simulink model "dynamik"  (R2016b)
settings: Solver=ode23s  StartTime=0.0  StopTime=100  RelTol=1e-3
values from neighbouring files (symbols this model uses):
  L = T-V    [modeldynamik.m]
undefined symbols (not defined in the file or in its folder): a_acc, a_de, dot_phi_soll, I_R, l, m, Mass
libraries: simulink x3
settings Model: Creator=Alexa  LastModifiedBy=Alexa

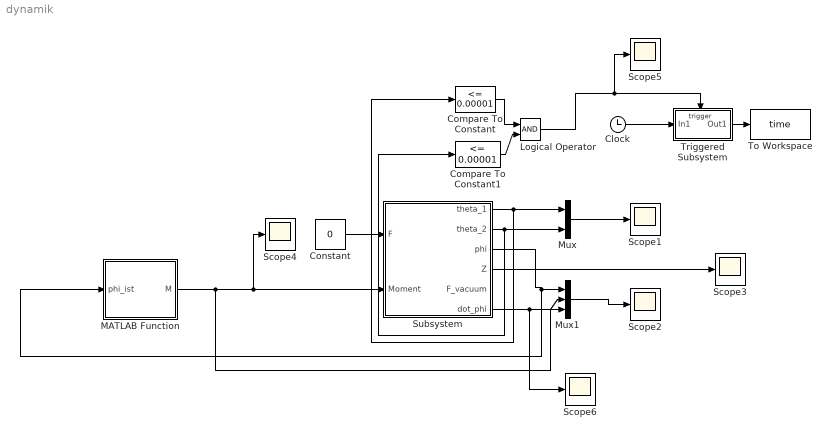
== system dynamik ==
  Clock : Clock
  Compare To Constant : simulink/Logic and Bit Operations/Compare To Constant  relop=<=  const=0.00001  OutDataTypeStr=boolean
  Compare To Constant1 : simulink/Logic and Bit Operations/Compare To Constant  relop=<=  const=0.00001  OutDataTypeStr=boolean
  Constant : Constant  Value=0
  Logical Operator : Logic  AllPortsSameDT=off  OutDataTypeStr=boolean
  MATLAB Function : MATLAB Function  TreatAsAtomicUnit=on
  Mux : Mux  Inputs=2
  Mux1 : Mux  Inputs=3
  Scope{1..6} (6 alike) : Scope
  Subsystem : Subsystem
  To Workspace : ToWorkspace  VariableName=time  SaveFormat=Timeseries  SampleTime=-1
  Triggered Subsystem : Subsystem  TreatAsAtomicUnit=on
  wires:
  Subsystem/1(theta_1) -> Compare To Constant/1, Mux/1
  Subsystem/2(theta_2) -> Compare To Constant1/1, Mux/2
  Mux/1 -> Scope1/1
  Subsystem/6(dot_phi) -> Scope6/1, Mux1/2
  Constant/1 -> Subsystem/1(F)
  Subsystem/3(phi) -> MATLAB Function/1(phi_ist), Mux1/1
  Mux1/1 -> Scope2/1
  Subsystem/4(Z) -> Scope3/1
  Clock/1 -> Triggered Subsystem/1(In1)
  Compare To Constant/1 -> Logical Operator/1
  Compare To Constant1/1 -> Logical Operator/2
  Logical Operator/1 -> Scope5/1, Triggered Subsystem/Trigger
  Triggered Subsystem/1(Out1) -> To Workspace/1
  MATLAB Function/1(M) -> Mux1/3, Subsystem/2(Moment), Scope4/1

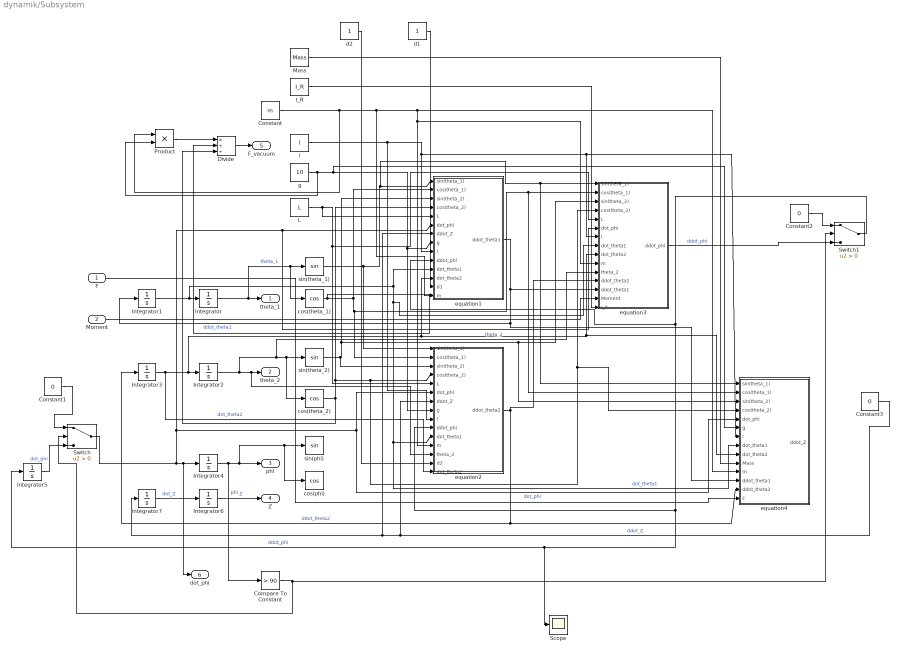
== system dynamik/Subsystem ==
  F : Inport
  Moment : Inport  Port=2
  Compare To Constant : simulink/Logic and Bit Operations/Compare To Constant  relop=>  const=90  OutDataTypeStr=boolean
  Constant : Constant  Value=m
  Constant1 : Constant  Value=0
  Constant2 : Constant  Value=0
  Constant3 : Constant  Value=0
  Divide : Product  Inputs=*//
  I_R : Constant  Value=I_R
  Integrator{,1..7} (8 alike) : Integrator
  L : Constant  Value=L
  Mass : Constant  Value=Mass
  Product : Product
  Scope : Scope
  Switch : Switch  Criteria=u2 > Threshold
  Switch1 : Switch  Criteria=u2 > Threshold
  cos(phi) : Trigonometry  Operator=cos
  cos(theta_1) : Trigonometry  Operator=cos
  cos(theta_2) : Trigonometry  Operator=cos
  d1 : Constant
  d2 : Constant
  equation1 : Subsystem
  equation2 : Subsystem
  equation3 : Subsystem
  equation4 : Subsystem
  g : Constant  Value=10
  l : Constant  Value=l
  sin(phi) : Trigonometry
  sin(theta_1) : Trigonometry
  sin(theta_2) : Trigonometry
  theta_1 : Outport
  theta_2 : Outport  Port=2
  phi : Outport  Port=3
  Z : Outport  Port=4
  F_vacuum : Outport  Port=5
  dot_phi : Outport  Port=6
  wires:
  Integrator/1 -> cos(theta_1)/1, sin(theta_1)/1, theta_1/1  "theta_1"
  Integrator1/1 -> equation1/11(dot_theta1), equation3/8(dot_theta1), equation4/8(dot_theta1), equation2/11(dot_theta1), Integrator/1  "dot_theta1"
  Integrator2/1 -> equation3/11(theta_2), cos(theta_2)/1, sin(theta_2)/1, equation2/13(theta_2), theta_2/1  "theta_2"
  Integrator3/1 -> equation2/15(dot_theta2), equation4/9(dot_theta2), equation3/9(dot_theta2), equation1/12(dot_theta2), Integrator2/1  "dot_theta2"
  Integrator4/1 -> Compare To Constant/1, cos(phi)/1, sin(phi)/1, phi/1  "phi"
  Integrator6/1 -> Z/1  "Z"
  Integrator7/1 -> Integrator6/1  "dot_Z"
  equation1/1(ddot_theta1) -> equation3/13(ddot_theta1), equation4/12(ddot_theta1), Integrator1/1  "ddot_theta1"
  equation2/1(ddot_theta2) -> equation3/12(ddot_theta2), equation4/13(ddot_theta2), Integrator3/1  "ddot_theta2"
  Constant3/1 -> equation1/7(ddot_Z), Integrator7/1, equation2/7(ddot_Z)  "ddot_Z"
  sin(theta_1)/1 -> equation2/1(sin(theta_1)), equation4/1(sin(theta_1)), equation3/1(sin(theta_1)), equation1/1(sin(theta_1))
  cos(theta_1)/1 -> Divide/2, equation2/2(cos(theta_1)), equation4/2(cos(theta_1)), equation3/2(cos(theta_1)), equation1/2(cos(theta_1))
  sin(theta_2)/1 -> equation2/3(sin(theta_2)), equation4/3(sin(theta_2)), equation3/3(sin(theta_2)), equation1/3(sin(theta_2))
  cos(theta_2)/1 -> Divide/3, equation4/4(cos(theta_2)), equation3/4(cos(theta_2)), equation2/4(cos(theta_2)), equation1/4(cos(theta_2))
  L/1 -> equation2/5(L), equation3/5(L), equation1/5(L)
  g/1 -> Product/2, equation4/6(g), equation2/8(g), equation1/8(g)
  l/1 -> equation2/9(l), equation4/7(l), equation3/7(l), equation1/9(l)
  Constant/1 -> Product/1, equation1/14(m), equation4/11(m), equation2/12(m), equation3/10(m)
  I_R/1 -> equation3/15(I_R)
  Mass/1 -> equation4/10(Mass)
  Product/1 -> Divide/1
  Divide/1 -> F_vacuum/1
  d1/1 -> equation1/13(d1)
  Moment/1 -> equation3/14(Moment)
  F/1 -> equation4/14(F)
  d2/1 -> equation2/14(d2)
  Switch/1 -> equation2/6(dot_phi), equation4/5(dot_phi), equation3/6(dot_phi), equation1/6(dot_phi), dot_phi/1, Integrator4/1  "dot_phi"
  Integrator5/1 -> Switch/3  "dot_phi"
  Compare To Constant/1 -> Switch/2, Switch1/2
  Constant1/1 -> Switch/1
  Switch1/1 -> equation1/10(ddot_phi), equation2/10(ddot_phi), Scope/1, Integrator5/1  "ddot_phi"
  Constant2/1 -> Switch1/1
  equation3/1(ddot_phi) -> Switch1/3  "ddot_phi"

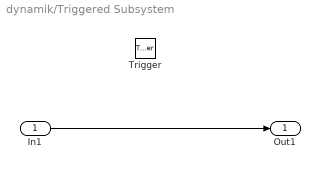
== system dynamik/Triggered Subsystem ==
  In1 : Inport
  Trigger : TriggerPort  VariantControl=Variant
  Out1 : Outport
  wires:
  In1/1 -> Out1/1

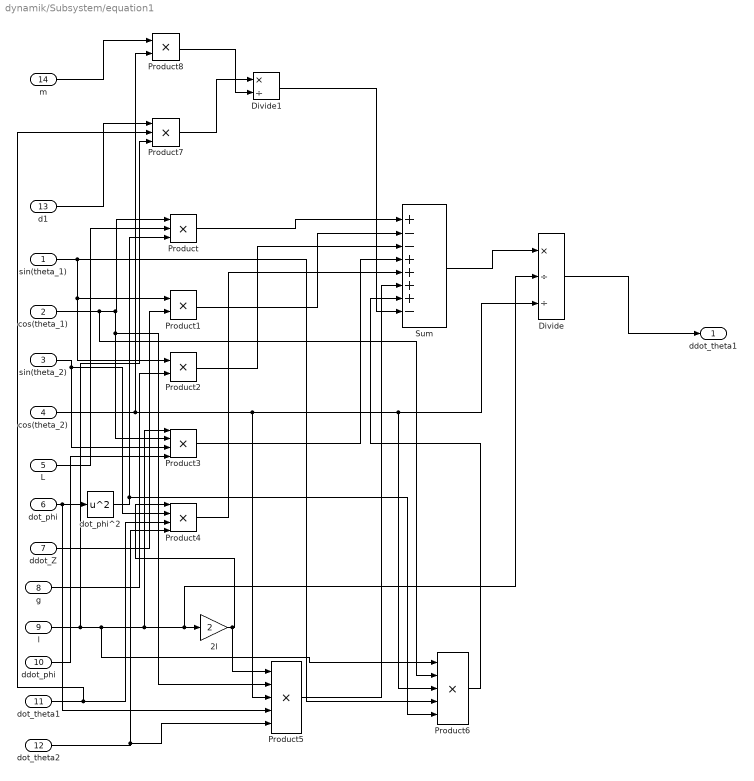
== system dynamik/Subsystem/equation1 ==
  sin(theta_1) : Inport
  cos(theta_1) : Inport  Port=2
  sin(theta_2) : Inport  Port=3
  cos(theta_2) : Inport  Port=4
  L : Inport  Port=5
  dot_phi : Inport  Port=6
  ddot_Z : Inport  Port=7
  g : Inport  Port=8
  l : Inport  Port=9
  ddot_phi : Inport  Port=10
  dot_theta1 : Inport  Port=11
  dot_theta2 : Inport  Port=12
  d1 : Inport  Port=13
  m : Inport  Port=14
  2l : Gain  Gain=2
  Divide : Product  Inputs=*//
  Divide1 : Product  Inputs=*/
  Product : Product  Inputs=3
  Product1 : Product
  Product2 : Product
  Product3 : Product  Inputs=4
  Product4 : Product  Inputs=4
  Product5 : Product  Inputs=5
  Product6 : Product  Inputs=5
  Product7 : Product  Inputs=3
  Product8 : Product
  Sum : Sum  Inputs=+--++++-
  dot_phi^2 : Math  Operator=square  SaturateOnIntegerOverflow=on
  ddot_theta1 : Outport
  wires:
  dot_phi/1 -> Product5/4, dot_phi^2/1
  cos(theta_1)/1 -> Product6/2, Product5/2, Product3/2, Product/1
  L/1 -> Product/2
  dot_phi^2/1 -> Product6/5, Product/3
  Product/1 -> Sum/1
  sin(theta_1)/1 -> Product6/4, Product2/1, Product1/1
  Product1/1 -> Sum/2
  ddot_Z/1 -> Product1/2
  g/1 -> Product2/2
  Product2/1 -> Sum/3
  l/1 -> Product7/3, Product6/1, Divide/2, 2l/1, Product3/1
  sin(theta_2)/1 -> Product4/2, Product3/3
  Product3/1 -> Sum/4
  ddot_phi/1 -> Product3/4
  2l/1 -> Product5/1, Product4/1
  dot_theta1/1 -> Product7/2, Product4/3
  dot_theta2/1 -> Product5/5, Product4/4
  Product4/1 -> Sum/5
  cos(theta_2)/1 -> Divide/3, Product6/3, Product5/3, Product8/2
  Product5/1 -> Sum/6
  Sum/1 -> Divide/1
  Product6/1 -> Sum/7
  Divide/1 -> ddot_theta1/1
  d1/1 -> Product7/1
  m/1 -> Product8/1
  Product7/1 -> Divide1/1
  Product8/1 -> Divide1/2
  Divide1/1 -> Sum/8

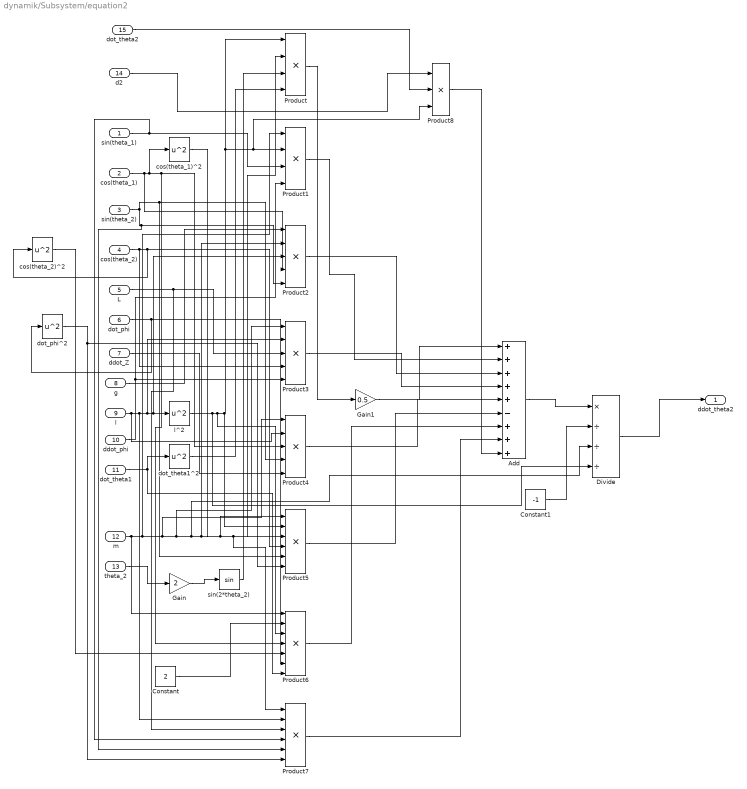
== system dynamik/Subsystem/equation2 ==
  sin(theta_1) : Inport
  cos(theta_1) : Inport  Port=2
  sin(theta_2) : Inport  Port=3
  cos(theta_2) : Inport  Port=4
  L : Inport  Port=5
  dot_phi : Inport  Port=6
  ddot_Z : Inport  Port=7
  g : Inport  Port=8
  l : Inport  Port=9
  ddot_phi : Inport  Port=10
  dot_theta1 : Inport  Port=11
  m : Inport  Port=12
  theta_2 : Inport  Port=13
  d2 : Inport  Port=14
  dot_theta2 : Inport  Port=15
  Add : Sum  Inputs=+++++-+++
  Constant : Constant  Value=2
  Constant1 : Constant  Value=-1
  Divide : Product  Inputs=*///
  Gain : Gain  Gain=2
  Gain1 : Gain  Gain=0.5
  Product : Product  Inputs=4
  Product1 : Product  Inputs=4
  Product2 : Product  Inputs=5
  Product3 : Product  Inputs=5
  Product4 : Product  Inputs=5
  Product5 : Product  Inputs=6
  Product6 : Product  Inputs=7
  Product7 : Product  Inputs=6
  Product8 : Product  Inputs=3
  cos(theta_1)^2 : Math  Operator=square  SaturateOnIntegerOverflow=on
  cos(theta_2)^2 : Math  Operator=square  SaturateOnIntegerOverflow=on
  dot_phi^2 : Math  Operator=square  SaturateOnIntegerOverflow=on
  dot_theta1^2 : Math  Operator=square  SaturateOnIntegerOverflow=on
  l^2 : Math  Operator=square  SaturateOnIntegerOverflow=on
  sin(2*theta_2) : Trigonometry
  ddot_theta2 : Outport
  wires:
  l/1 -> Product4/2, Product7/2, Product3/2, Product2/3, l^2/1
  l^2/1 -> Divide/4, Product6/3, Product5/2, Product/1, Product8/3, Product1/2
  m/1 -> Product6/1, Product1/1, Product4/1, Product3/1, Divide/3, Product2/2, Product5/1, Product/2
  theta_2/1 -> Gain/1
  Gain/1 -> sin(2*theta_2)/1
  sin(2*theta_2)/1 -> Product/3
  dot_theta1/1 -> Product6/7, dot_theta1^2/1
  dot_theta1^2/1 -> Product/4
  Product/1 -> Gain1/1
  Gain1/1 -> Add/1
  sin(theta_1)/1 -> Product7/4, Product1/3
  ddot_phi/1 -> Product1/4, Product3/5
  Product1/1 -> Add/2
  g/1 -> Product2/1
  cos(theta_1)/1 -> cos(theta_1)^2/1, Product6/4, Product4/3, Product2/4
  sin(theta_2)/1 -> Product7/5, Product2/5, Product5/5, Product4/4
  Product2/1 -> Add/3
  L/1 -> Product7/3, Product3/3
  cos(theta_2)/1 -> cos(theta_2)^2/1, Product5/4, Product3/4
  Product3/1 -> Add/4
  ddot_Z/1 -> Product4/5
  Product4/1 -> Add/5
  cos(theta_1)^2/1 -> Product7/1, Product5/3
  dot_phi/1 -> Product6/6, dot_phi^2/1
  dot_phi^2/1 -> Product7/6, Product5/6
  Product5/1 -> Add/6
  Constant/1 -> Product6/2
  cos(theta_2)^2/1 -> Product6/5
  Product6/1 -> Add/7
  Product7/1 -> Add/8
  Add/1 -> Divide/1
  Constant1/1 -> Divide/2
  Divide/1 -> ddot_theta2/1
  d2/1 -> Product8/1
  dot_theta2/1 -> Product8/2
  Product8/1 -> Add/9

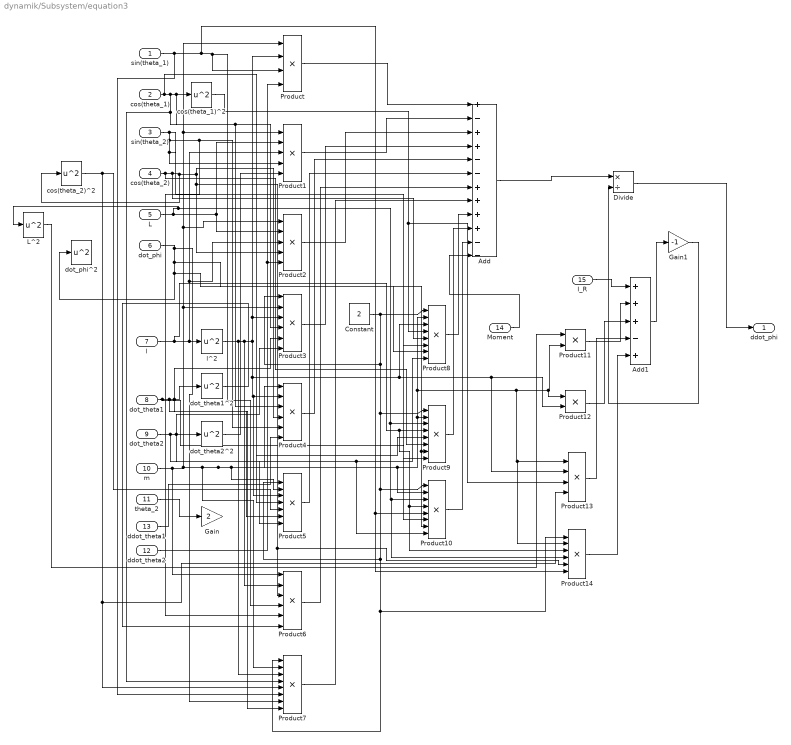
== system dynamik/Subsystem/equation3 ==
  sin(theta_1) : Inport
  cos(theta_1) : Inport  Port=2
  sin(theta_2) : Inport  Port=3
  cos(theta_2) : Inport  Port=4
  L : Inport  Port=5
  dot_phi : Inport  Port=6
  l : Inport  Port=7
  dot_theta1 : Inport  Port=8
  dot_theta2 : Inport  Port=9
  m : Inport  Port=10
  theta_2 : Inport  Port=11
  ddot_theta2 : Inport  Port=12
  ddot_theta1 : Inport  Port=13
  Moment : Inport  Port=14
  I_R : Inport  Port=15
  Add : Sum  Inputs=+-++--++++--
  Add1 : Sum  Inputs=+++-+
  Constant : Constant  Value=2
  Divide : Product  Inputs=*/
  Gain : Gain  Gain=2
  Gain1 : Gain  Gain=-1
  L^2 : Math  Operator=square  SaturateOnIntegerOverflow=on
  Product : Product  Inputs=4
  Product1 : Product  Inputs=5
  Product{7..10} (4 alike) : Product  Inputs=8
  Product11 : Product
  Product12 : Product
  Product13 : Product  Inputs=4
  Product{3..4,6,14} (4 alike) : Product  Inputs=6
  Product2 : Product  Inputs=5
  Product5 : Product  Inputs=7
  cos(theta_1)^2 : Math  Operator=square  SaturateOnIntegerOverflow=on
  cos(theta_2)^2 : Math  Operator=square  SaturateOnIntegerOverflow=on
  dot_phi^2 : Math  Operator=square  SaturateOnIntegerOverflow=on
  dot_theta1^2 : Math  Operator=square  SaturateOnIntegerOverflow=on
  dot_theta2^2 : Math  Operator=square  SaturateOnIntegerOverflow=on
  l^2 : Math  Operator=square  SaturateOnIntegerOverflow=on
  ddot_phi : Outport
  wires:
  l/1 -> Product14/3, Product10/4, Product9/4, Product2/3, Product1/3, l^2/1
  theta_2/1 -> Gain/1
  dot_theta1/1 -> Product9/8, Product7/8, Product5/6, Product3/5, dot_theta1^2/1
  cos(theta_1)/1 -> Product9/5, Product7/4, Product5/4, Product4/3, Product3/4, cos(theta_1)^2/1
  cos(theta_2)/1 -> Product9/6, Product8/5, Product4/4, Product14/5, Product6/3, Product2/4, cos(theta_2)^2/1
  dot_phi/1 -> Product7/7, Product8/7, Product10/7, Product9/7, dot_phi^2/1
  m/1 -> Product6/1, Product7/2, Product10/2, Product9/2, Product14/2, Product13/1, Product12/1, Product11/2, Product8/2, Product5/2, Product4/1, Product3/2, Product2/1, Product1/1, Product/1
  sin(theta_1)/1 -> Product7/6, Product14/6, Product10/5, Product6/4, Product/3
  ddot_theta2/1 -> Product2/5, Product/4
  Product/1 -> Add/1
  L/1 -> L^2/1, Product14/4, Product10/3, Product9/3, Product2/2, Product1/2
  sin(theta_2)/1 -> Product10/6, Product6/5, Product4/5, Product8/6, Product1/4
  dot_theta2^2/1 -> Product1/5
  Product1/1 -> Add/2
  Product2/1 -> Add/3
  Constant/1 -> Product8/1, Product9/1, Product10/1, Product14/1, Product7/1, Product5/1, Product3/1
  Product3/1 -> Add/4
  ddot_theta1/1 -> Product4/6
  Product4/1 -> Add/5
  cos(theta_2)^2/1 -> Product13/4, Product7/5, Product5/5
  Product5/1 -> Add/6
  dot_theta1^2/1 -> Product6/6
  Product6/1 -> Add/7
  Product7/1 -> Add/8
  cos(theta_1)^2/1 -> Product13/3, Product8/4
  Product8/1 -> Add/9
  Product9/1 -> Add/10
  dot_theta2/1 -> Product10/8, Product8/8, Product5/7, Product3/6, dot_theta2^2/1
  Product10/1 -> Add/11
  Moment/1 -> Add/12
  I_R/1 -> Add1/1
  Product11/1 -> Add1/2
  L^2/1 -> Product11/1
  l^2/1 -> Product7/3, Product6/2, Product13/2, Product12/2, Product8/3, Product5/3, Product4/2, Product3/3, Product/2
  Product12/1 -> Add1/3
  Product13/1 -> Add1/4
  Product14/1 -> Add1/5
  Add1/1 -> Gain1/1
  Gain1/1 -> Divide/2
  Add/1 -> Divide/1
  Divide/1 -> ddot_phi/1

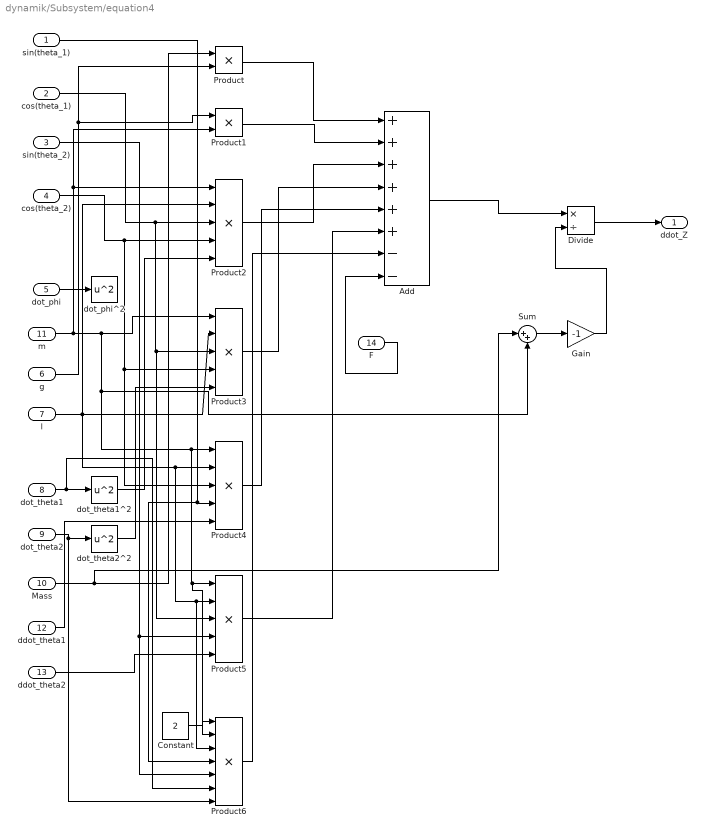
== system dynamik/Subsystem/equation4 ==
  sin(theta_1) : Inport
  cos(theta_1) : Inport  Port=2
  sin(theta_2) : Inport  Port=3
  cos(theta_2) : Inport  Port=4
  dot_phi : Inport  Port=5
  g : Inport  Port=6
  l : Inport  Port=7
  dot_theta1 : Inport  Port=8
  dot_theta2 : Inport  Port=9
  Mass : Inport  Port=10
  m : Inport  Port=11
  ddot_theta1 : Inport  Port=12
  ddot_theta2 : Inport  Port=13
  F : Inport  Port=14
  Add : Sum  Inputs=++++++--
  Constant : Constant  Value=2
  Divide : Product  Inputs=*/
  Gain : Gain  Gain=-1
  Product : Product
  Product1 : Product
  Product{2..5} (4 alike) : Product  Inputs=5
  Product6 : Product  Inputs=7
  Sum : Sum  Inputs=|++
  dot_phi^2 : Math  Operator=square  SaturateOnIntegerOverflow=on
  dot_theta1^2 : Math  Operator=square  SaturateOnIntegerOverflow=on
  dot_theta2^2 : Math  Operator=square  SaturateOnIntegerOverflow=on
  ddot_Z : Outport
  wires:
  dot_phi/1 -> dot_phi^2/1
  Mass/1 -> Sum/1, Product/1
  g/1 -> Product1/1, Product/2
  Product/1 -> Add/1
  m/1 -> Sum/2, Product6/2, Product5/1, Product4/1, Product3/1, Product2/1, Product1/2
  Product1/1 -> Add/2
  l/1 -> Product6/3, Product5/2, Product4/2, Product3/2, Product2/2
  cos(theta_1)/1 -> Product5/3, Product3/3, Product2/3
  cos(theta_2)/1 -> Product4/3, Product3/4, Product2/4
  dot_theta1/1 -> Product6/6, dot_theta1^2/1
  dot_theta1^2/1 -> Product2/5
  Product2/1 -> Add/3
  dot_theta2/1 -> Product6/7, dot_theta2^2/1
  dot_theta2^2/1 -> Product3/5
  Product3/1 -> Add/4
  sin(theta_1)/1 -> Product6/4, Product4/4
  ddot_theta1/1 -> Product4/5
  Product4/1 -> Add/5
  sin(theta_2)/1 -> Product6/5, Product5/4
  ddot_theta2/1 -> Product5/5
  Product5/1 -> Add/6
  Constant/1 -> Product6/1
  Product6/1 -> Add/7
  F/1 -> Add/8
  Add/1 -> Divide/1
  Sum/1 -> Gain/1
  Gain/1 -> Divide/2
  Divide/1 -> ddot_Z/1

== matlab function dynamik/MATLAB Function ==
  data: M output; a_acc parameter; I_R parameter; dot_phi_soll parameter; phi_ist input; a_de parameter
function M = fcn(a_acc,I_R, dot_phi_soll,phi_ist, a_de)
L_1=(0.5*dot_phi_soll^2/a_acc); % rad 
L_2=(90-0.5*dot_phi_soll^2/a_de); % rad
  if phi_ist<=L_1 % Drift Fehler
     M=I_R*a_acc+10;
  else if phi_ist>=L_2&&phi_ist<90
     M=-I_R*a_de;
  else
     M=0;
  end
 end
